simulink model "Modelisation_1"  (R2016a)
settings: Solver=VariableStepAuto  StartTime=0.0  StopTime=10  RelTol=1e-3
undefined symbols (not defined in the file or in its folder): augstate, csys, K, N
libraries: simulink x12, cstblocks x3
settings Model: Creator=Ludwig  LastModifiedBy=Ludwig

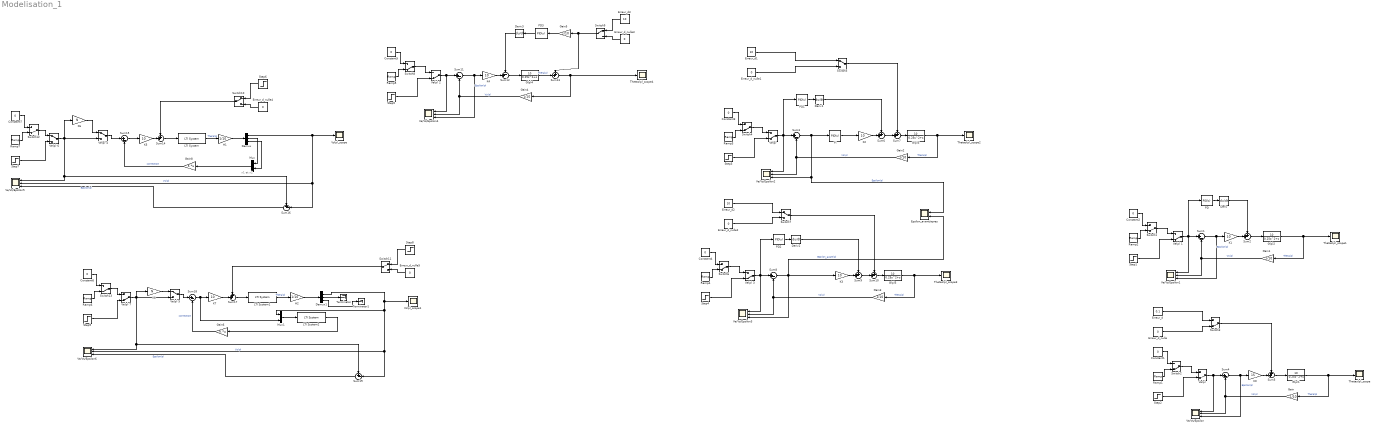
== system Modelisation_1 ==
  note: x1 et x2
  Constant{1..7} (7 alike) : Constant  Value=0
  Demux : Demux  Outputs=3
  Demux1 : Demux  Outputs=3
  Deriv{,1..3} (4 alike) : Derivative
  Epsilon_avant/apres : Scope  NumInputPorts=2
  Erreur_d : Constant  Value=0.1
  Erreur_d1 : Constant  Value=10
  Erreur_d2 : Constant  Value=10
  Erreur_d3 : Constant  Value=10
  Erreur_d_nulle{,1..5} (6 alike) : Constant  Value=0
  G(p){1..5} (5 alike) : TransferFcn  Numerator=[10]  Denominator=[0.25 1 0]
  Gain{,1..5} (6 alike) : Gain  Gain=1/10
  Gain6 : Gain  Gain=K  Multiplication=Matrix(K*u)
  Gain8 : Gain  Gain=K  Multiplication=Matrix(K*u)
  H1 : Gain  Gain=1/10
  H2 : Gain  Gain=1/10
  K0 : Gain  Gain=15
  K{1..5,7} (6 alike) : Gain  Gain=10
  K6 : Gain  Gain=N
  K8 : Gain  Gain=N
  LTI System : cstblocks/LTI System  sys=augstate(csys)  IC=[]
  LTI System1 : cstblocks/LTI System  sys=augstate(csys)  IC=[]
  LTI System2 : cstblocks/LTI System  sys=sys_obs  IC=[]
  Mux : Mux  Inputs=2
  Mux1 : Mux  Inputs=2
  PD{,1..3} (4 alike) : simulink/Continuous/PID Controller  Controller=PID  TimeDomain=Continuous-time  SampleTime=-1  IntegratorMethod=Forward Euler  FilterMethod=Forward Euler  Form=Parallel  UseFilter=on  ControllerParametersSource=internal  P=1  I=0  D=0.25  N=100  InitialConditionSource=internal  InitialConditionForIntegrator=0  InitialConditionForFilter=0  ExternalReset=none  LimitOutput=off  UpperSaturationLimit=inf  LowerSaturationLimit=-inf  LinearizeAsGain=on  AntiWindupMode=none  Kb=1  TrackingMode=off  Kt=1  PParamMin=[]  PParamMax=[]  IParamMin=[]  IParamMax=[]  DParamMin=[]  DParamMax=[]  NParamMin=[]  NParamMax=[]  KbParamMin=[]  KbParamMax=[]  KtParamMin=[]  KtParamMax=[]  POutMin=[]  POutMax=[]  IOutMin=[]  IOutMax=[]  DOutMin=[]  DOutMax=[]  NOutMin=[]  NOutMax=[]  KbOutMin=[]  KbOutMax=[]  KtOutMin=[]  KtOutMax=[]  IntegratorOutMin=[]  IntegratorOutMax=[]  FilterOutMin=[]  FilterOutMax=[]  SumOutMin=[]  SumOutMax=[]  SumI1OutMin=[]  SumI1OutMax=[]  SumI2OutMin=[]  SumI2OutMax=[]  SumI3OutMin=[]  SumI3OutMax=[]  SumDOutMin=[]  SumDOutMax=[]  SaturationOutMin=[]  SaturationOutMax=[]  IntegratorContinuousStateAttributes=''  IntegratorStateMustResolveToSignalObject=off  IntegratorRTWStateStorageClass=Auto  FilterContinuousStateAttributes=''  FilterStateMustResolveToSignalObject=off  FilterRTWStateStorageClass=Auto  DifferentiatorICPrevScaledInput=0  DifferentiatorOutMin=[]  DifferentiatorOutMax=[]
  Pi : simulink/Continuous/PID Controller  Controller=PID  TimeDomain=Continuous-time  SampleTime=-1  IntegratorMethod=Forward Euler  FilterMethod=Forward Euler  Form=Parallel  UseFilter=on  ControllerParametersSource=internal  P=1  I=1  D=0  N=100  InitialConditionSource=internal  InitialConditionForIntegrator=0  InitialConditionForFilter=0  ExternalReset=none  LimitOutput=off  UpperSaturationLimit=inf  LowerSaturationLimit=-inf  LinearizeAsGain=on  AntiWindupMode=none  Kb=1  TrackingMode=off  Kt=1  PParamMin=[]  PParamMax=[]  IParamMin=[]  IParamMax=[]  DParamMin=[]  DParamMax=[]  NParamMin=[]  NParamMax=[]  KbParamMin=[]  KbParamMax=[]  KtParamMin=[]  KtParamMax=[]  POutMin=[]  POutMax=[]  IOutMin=[]  IOutMax=[]  DOutMin=[]  DOutMax=[]  NOutMin=[]  NOutMax=[]  KbOutMin=[]  KbOutMax=[]  KtOutMin=[]  KtOutMax=[]  IntegratorOutMin=[]  IntegratorOutMax=[]  FilterOutMin=[]  FilterOutMax=[]  SumOutMin=[]  SumOutMax=[]  SumI1OutMin=[]  SumI1OutMax=[]  SumI2OutMin=[]  SumI2OutMax=[]  SumI3OutMin=[]  SumI3OutMax=[]  SumDOutMin=[]  SumDOutMax=[]  SaturationOutMin=[]  SaturationOutMax=[]  IntegratorContinuousStateAttributes=''  IntegratorStateMustResolveToSignalObject=off  IntegratorRTWStateStorageClass=Auto  FilterContinuousStateAttributes=''  FilterStateMustResolveToSignalObject=off  FilterRTWStateStorageClass=Auto  DifferentiatorICPrevScaledInput=0  DifferentiatorOutMin=[]  DifferentiatorOutMax=[]
  Ramp{1..7} (7 alike) : simulink/Sources/Ramp  slope=1  start=0  X0=0
  Step{1..5,7,9} (7 alike) : Step  SampleTime=0
  Step6 : Step  After=10  SampleTime=0
  Step8 : Step  After=10  SampleTime=0
  Sum{1,3..4,8,11,15,18} (7 alike) : Sum  Inputs=|+-
  Sum{2,5..7,9..10,13..14,17} (9 alike) : Sum  Inputs=++|
  Sum12 : Sum  Inputs=-+|
  Sum16 : Sum  Inputs=+-|
  Sum19 : Sum  Inputs=+-|
  Switch{1..4,6,8,12..13} (8 alike) : ManualSwitch  CurrentSetting=0
  Switch{5,7,9..11} (5 alike) : ManualSwitch
  Terminator : Terminator
  Terminator1 : Terminator
  Thetas(p)_scope{,1..4} (5 alike) : Scope
  Ve(p) {,,1..3,7} (6 alike) : ManualSwitch  CurrentSetting=0
  Ve(p) 4 : ManualSwitch
  Ve(p) 5 : ManualSwitch
  Ve(p) 6 : ManualSwitch
  Ve/Vs/Epsilon{,1..6} (7 alike) : Scope  NumInputPorts=3
  Vs(p)_scope : Scope
  Vs(p)_scope1 : Scope
  wires:
  Constant1/1 -> Switch2/1
  Ramp1/1 -> Switch2/2
  Erreur_d/1 -> Switch3/1
  Erreur_d_nulle/1 -> Switch3/2
  Sum4/1 -> Ve/Vs/Epsilon/3, K0/1  "Epsilon(p)"
  Switch3/1 -> Sum5/1
  Sum5/1 -> G(p)1/1
  G(p)1/1 -> Gain/1, Thetas(p)_scope/1  "Thera(p)"
  Gain/1 -> Ve/Vs/Epsilon/2, Sum4/2  "Vs(p)"
  Step2/1 -> "Ve(p) "/2
  Switch2/1 -> "Ve(p) "/1
  "Ve(p) "/1 -> Ve/Vs/Epsilon/1, Sum4/1
  K0/1 -> Sum5/2
  Constant2/1 -> Switch1/1
  Ramp2/1 -> Switch1/2
  Sum1/1 -> Ve/Vs/Epsilon1/3, K1/1  "Epsilon(p)"
  Sum2/1 -> G(p)2/1
  G(p)2/1 -> Gain1/1, Thetas(p)_scope1/1  "Thera(p)"
  Gain1/1 -> Ve/Vs/Epsilon1/2, Sum1/2  "Vs(p)"
  Step1/1 -> Ve(p) 1/2
  Switch1/1 -> Ve(p) 1/1
  Ve(p) 1/1 -> PD/1, Ve/Vs/Epsilon1/1, Sum1/1
  K1/1 -> Sum2/2
  Deriv/1 -> Sum2/1
  PD/1 -> Deriv/1
  Constant3/1 -> Switch4/1
  Ramp3/1 -> Switch4/2
  Sum3/1 -> Pi/1, Epsilon_avant/apres/1, Ve/Vs/Epsilon2/3  "Epsilon(p)"
  G(p)3/1 -> Gain2/1, Thetas(p)_scope2/1  "Thera(p)"
  Gain2/1 -> Ve/Vs/Epsilon2/2, Sum3/2  "Vs(p)"
  Step3/1 -> "Ve(p) "/2
  Switch4/1 -> "Ve(p) "/1
  "Ve(p) "/1 -> PD1/1, Ve/Vs/Epsilon2/1, Sum3/1
  K2/1 -> Sum6/2
  Deriv1/1 -> Sum6/1
  PD1/1 -> Deriv1/1
  Erreur_d1/1 -> Switch5/1
  Erreur_d_nulle1/1 -> Switch5/2
  Switch5/1 -> Sum7/1
  Sum7/1 -> G(p)3/1
  Sum6/1 -> Sum7/2
  Constant4/1 -> Switch6/1
  Ramp4/1 -> Switch6/2
  Sum8/1 -> Epsilon_avant/apres/2, K3/1, Ve/Vs/Epsilon3/3  "Epsilon_avant(p)"
  G(p)5/1 -> Gain3/1, Thetas(p)_scope3/1  "Thera(p)"
  Gain3/1 -> Ve/Vs/Epsilon3/2, Sum8/2  "Vs(p)"
  Step4/1 -> Ve(p) 3/2
  Switch6/1 -> Ve(p) 3/1
  Ve(p) 3/1 -> PD2/1, Ve/Vs/Epsilon3/1, Sum8/1
  K3/1 -> Sum9/2
  Deriv2/1 -> Sum9/1
  PD2/1 -> Deriv2/1
  Erreur_d2/1 -> Switch7/1
  Erreur_d_nulle2/1 -> Switch7/2
  Switch7/1 -> Sum10/1
  Sum10/1 -> G(p)5/1
  Sum9/1 -> Sum10/2
  Pi/1 -> K2/1
  Constant5/1 -> Switch8/1
  Ramp5/1 -> Switch8/2
  Sum11/1 -> Ve/Vs/Epsilon4/3, K4/1  "Epsilon(p)"
  Sum12/1 -> G(p)4/1
  Gain4/1 -> Ve/Vs/Epsilon4/2, Sum11/2  "Vs(p)"
  Step5/1 -> Ve(p) 2/2
  Switch8/1 -> Ve(p) 2/1
  Ve(p) 2/1 -> Ve/Vs/Epsilon4/1, Sum11/1
  K4/1 -> Sum12/2
  PD3/1 -> Deriv3/1
  Erreur_d3/1 -> Switch9/1
  Erreur_d_nulle3/1 -> Switch9/2
  Switch9/1 -> Gain5/1, Sum13/1
  G(p)4/1 -> Sum13/2  "Thera(p)"
  Sum13/1 -> Thetas(p)_scope4/1, Gain4/1
  Deriv3/1 -> Sum12/1
  Gain5/1 -> PD3/1
  Constant7/1 -> Switch12/1
  Ramp7/1 -> Switch12/2
  Sum15/1 -> K5/1
  Step7/1 -> Ve(p) 6/2
  Switch12/1 -> Ve(p) 6/1
  Ve(p) 6/1 -> Sum16/1, Ve/Vs/Epsilon5/1, Ve(p) 4/2, K6/1
  LTI System/1 -> H1/1  "Thera(p)"
  Mux/1 -> Gain8/1
  Demux/2 -> Mux/1
  Demux/3 -> Mux/2
  Step6/1 -> Switch10/1
  Erreur_d_nulle4/1 -> Switch10/2
  K5/1 -> Sum14/2
  Sum14/1 -> LTI System/1
  Switch10/1 -> Sum14/1
  K6/1 -> Ve(p) 4/1
  Ve(p) 4/1 -> Sum15/1
  Gain8/1 -> Sum15/2  "correctioin"
  Demux/1 -> Ve/Vs/Epsilon5/2, Sum16/2, Vs(p)_scope/1  "Vs(p)"
  H1/1 -> Demux/1
  Sum16/1 -> Ve/Vs/Epsilon5/3  "Epsilon(p)"
  Constant6/1 -> Switch13/1
  Ramp6/1 -> Switch13/2
  Sum18/1 -> Mux1/2, K7/1
  Step9/1 -> Ve(p) 7/2
  Switch13/1 -> Ve(p) 7/1
  Ve(p) 7/1 -> Sum19/1, Ve/Vs/Epsilon6/1, Ve(p) 5/2, K8/1
  LTI System1/1 -> H2/1  "Thera(p)"
  Step8/1 -> Switch11/1
  Erreur_d_nulle5/1 -> Switch11/2
  K7/1 -> Sum17/2
  Sum17/1 -> LTI System1/1
  Switch11/1 -> Sum17/1
  K8/1 -> Ve(p) 5/1
  Ve(p) 5/1 -> Sum18/1
  Gain6/1 -> Sum18/2  "correctioin"
  Demux1/1 -> Ve/Vs/Epsilon6/2, Sum19/2, Mux1/1, Vs(p)_scope1/1  "Vs(p)"
  H2/1 -> Demux1/1
  Sum19/1 -> Ve/Vs/Epsilon6/3  "Epsilon(p)"
  Demux1/2 -> Terminator/1
  Demux1/3 -> Terminator1/1
  Mux1/1 -> LTI System2/1
  LTI System2/1 -> Gain6/1
